simulink model "Jacobian"  (R2017b)
settings: Solver=VariableStepAuto  StartTime=0.0  StopTime=10.0  RelTol=1e-3
settings Model: Creator=Kalana  LastModifiedBy=Kalana

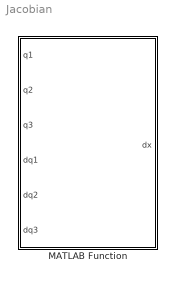
== system Jacobian ==
  MATLAB Function : MATLAB Function  TreatAsAtomicUnit=on

== matlab function Jacobian/MATLAB Function ==
  data: q1 input; dx output; q2 input; q3 input; dq1 input; dq2 input; dq3 input
function dx = Jacobian(q1, q2, q3, dq1, dq2, dq3)

dq = [ dq1;
       dq2;
       dq3];

JvEE =[-0.265*sind(q1)*cosd(q2-q3)-0.2*sind(q1)*cosd(q2)-0.1225*sind(q1)-0.0525*cosd(q1), -0.265*cosd(q1)*sind(q2-q3)-0.2*cosd(q1)*sind(q2),     0.265*cosd(q1)*sind(q2-q3) ;
       0,                                                                                 0.265*cosd(q2-q3)+0.2*cosd(q2),                        -0.265*cosd(q2-q3)         ;
       -0.265*cosd(q1)*cosd(q2-q3)-0.2*cosd(q1)*cosd(q2)-0.1225*cosd(q1)+0.0525*sind(q1), 0.265*sind(q1)*sind(q2-q3)+0.2*sind(q1)*sind(q2),      -0.265*sind(q1)*sind(q2-q3)]; 
   
dx = JvEE*dq;
